simulink model "OnePhInverterRL_17b"  (R2020a)
settings: Solver=ode23tb  StartTime=0.0  StopTime=1  MaxStep=2e-3  RelTol=1e-3
model workspace (MAT data in the model file):
  TLoad = [0.005 0.1]
libraries: powerlib x15, powerlib_meascontrol x9
settings Model: Creator=theo  LastModifiedBy=Theodore
settings DebuggingCC: ArithmeticOperatorsInVariantConditions=warning
settings SFSimCC: CustomCodeUndefinedFunction=UseInterfaceOnly

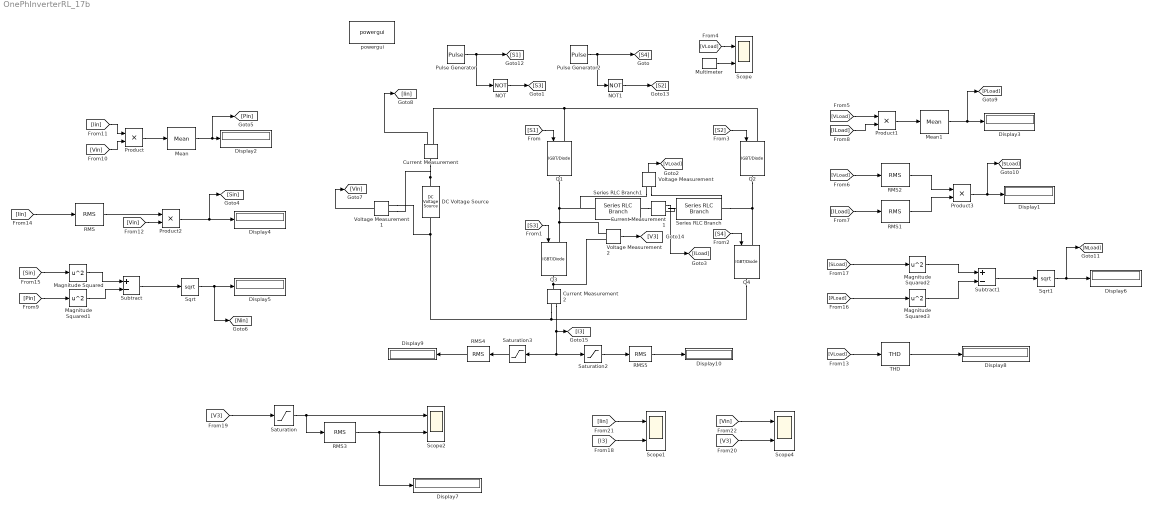
== system OnePhInverterRL_17b ==
  Current Measurement : powerlib/Measurements/Current Measurement  PhasorSimulation=off  OutputType=Complex  PSBequivalent=0
  Current Measurement1 : powerlib/Measurements/Current Measurement  PhasorSimulation=off  OutputType=Complex  PSBequivalent=0
  Current Measurement2 : powerlib/Measurements/Current Measurement  PhasorSimulation=off  OutputType=Complex  PSBequivalent=0
  DC Voltage Source : powerlib/Electrical Sources/DC Voltage Source  Amplitude=537.97  Measurements=None
  Display{1..10} (10 alike) : Display
  Magnitude Squared{,1..3} (4 alike) : Math  Operator=square  SaturateOnIntegerOverflow=on
  Mean : powerlib_meascontrol/Measurements/Mean  Freq=50  Vinit=0  Ts=0
  Mean1 : powerlib_meascontrol/Measurements/Mean  Freq=50  Vinit=0  Ts=0
  Multimeter : powerlib/Measurements/Multimeter  PhasorSimulation=off  OutputType=Complex  sel=2  L=2  Gain=1  yselected={'Ib: Series RLC Branch1'};  PSBOutputType=1  PSBequivalent=0  AxesSetting=[0,0.1,-100,100]  Display=0  SavedBlockNames=-11
  NOT : Logic  Operator=NOT  IconShape=distinctive  AllPortsSameDT=off  OutDataTypeStr=boolean
  NOT1 : Logic  Operator=NOT  IconShape=distinctive  AllPortsSameDT=off  OutDataTypeStr=boolean
  Product{,1..3} (4 alike) : Product
  Pulse Generator : DiscretePulseGenerator  PulseType=Time based  Period=0.02  PulseWidth=50
  Pulse Generator2 : DiscretePulseGenerator  PulseType=Time based  Period=0.02  PulseWidth=50
  Q{1..4} (4 alike) : powerlib/Power Electronics/IGBT//Diode  Ron=1e-3  Rs=1e5  Cs=inf  Measurements=off
  RMS{,1..5} (6 alike) : powerlib_meascontrol/Measurements/RMS  TrueRMS=on  Freq=50  RMSInit=120  Ts=0
  Saturation : Saturate  UpperLimit=0  LowerLimit=-50
  Saturation2 : Saturate  UpperLimit=0  LowerLimit=-100
  Saturation3 : Saturate  UpperLimit=100  LowerLimit=0
  Scope{,1..2,4} (4 alike) : Scope  NumInputPorts=2
  Series RLC Branch : powerlib/Elements/Series RLC Branch  LConnTagsString=__new0  RConnTagsString=__new0  BranchType=L  Resistance=10  Inductance=1/(2*pi)  SetiL0=off  InitialCurrent=0  Capacitance=1e-6  Setx0=off  InitialVoltage=0  Measurements=None
  Series RLC Branch1 : powerlib/Elements/Series RLC Branch  LConnTagsString=__new0  RConnTagsString=__new0  BranchType=R  Resistance=50  Inductance=1e-3  SetiL0=off  InitialCurrent=0  Capacitance=1e-6  Setx0=off  InitialVoltage=0  Measurements=Branch voltage and current
  Sqrt : Sqrt  SaturateOnIntegerOverflow=on
  Sqrt1 : Sqrt  SaturateOnIntegerOverflow=on
  Subtract : Sum  Inputs=+-
  Subtract1 : Sum  Inputs=+-
  THD : powerlib_meascontrol/Measurements/THD  Freq=50  Ts=0
  Voltage Measurement : powerlib/Measurements/Voltage Measurement  PhasorSimulation=off  OutputType=Complex  PSBequivalent=0
  Voltage Measurement1 : powerlib/Measurements/Voltage Measurement  PhasorSimulation=off  OutputType=Complex  PSBequivalent=0
  Voltage Measurement2 : powerlib/Measurements/Voltage Measurement  PhasorSimulation=off  OutputType=Complex  PSBequivalent=0
  powergui : powerlib/powergui  Priority=1  SimulationMode=Continuous  SampleTime=50e-6  frequency=50  Iterations=50  frequencyindice=0  Pbase=100e6  ErrMax=1e-4  UnitsV=kV  UnitsW=MW  buscounter=0  FunctionMessages=off  echomessages=off  EnableUseOfTLC=off  CurrentSourceSwitches=off  DisableSnubberDevices=on  DisableRonSwitches=on  DisableVfSwitches=on  DisplayEquations=off  AutomaticDiscreteSolvers=off  SolverType=Tustin/Backward Euler (TBE)  Interpol=off  ExternalGateDelay=off  methode=off  Ts=100  x0status=blocks  SPID=on  SwTol=0  HookPort=off  NonlinearTolerance=1e-4  nMaxIteration=100  ContinueOnMaxIteration=off  RestoreLinks=warning  ResistiveCurrentMeasurement=off  Frange=[0:2:500]  Ylog=off  Xlog=on  ShowGrid=off  save=off  variable=ZData  structure=0  ZoomFFT=off  StartTime=0.0  cycles=1  DisplayStyle=1  fundamental=60  FreqAxis=off  MaxFrequency=1000  frequencyindicesteady=1  RmsSteady=1  display=off
  wires:
  Pulse Generator/1 -> NOT/1, [S1]
  NOT/1 -> [S3]
  [S1] -> Q1/1
  [S4] -> Q4/1
  [S3] -> Q3/1
  [S2] -> Q2/1
  Voltage Measurement/1 -> [VLoad]
  [VLoad] -> Scope/1
  Multimeter/1 -> Scope/2
  Current Measurement/1 -> [Iin]
  Product/1 -> Mean/1
  Mean/1 -> [Pin], Display2/1
  Voltage Measurement1/1 -> [Vin]
  [VLoad] -> Product1/1
  Product1/1 -> Mean1/1
  Mean1/1 -> [PLoad], Display3/1
  RMS/1 -> Product2/1
  Product2/1 -> [Sin], Display4/1
  RMS2/1 -> Product3/1
  RMS1/1 -> Product3/2
  Current Measurement1/1 -> [ILoad]
  [ILoad] -> RMS1/1
  [VLoad] -> RMS2/1
  [ILoad] -> Product1/2
  Magnitude Squared/1 -> Subtract/1
  Magnitude Squared1/1 -> Subtract/2
  Subtract/1 -> Sqrt/1
  Sqrt/1 -> [Nin], Display5/1
  Subtract1/1 -> Sqrt1/1
  Product3/1 -> [SLoad], Display1/1
  Magnitude Squared2/1 -> Subtract1/1
  Magnitude Squared3/1 -> Subtract1/2
  Sqrt1/1 -> [NLoad], Display6/1
  [Vin] -> Product/2
  [Vin] -> Product2/2
  [Iin] -> Product/1
  [Iin] -> RMS/1
  [Pin] -> Magnitude Squared1/1
  [Sin] -> Magnitude Squared/1
  [PLoad] -> Magnitude Squared3/1
  [SLoad] -> Magnitude Squared2/1
  Pulse Generator2/1 -> [S4], NOT1/1
  NOT1/1 -> [S2]
  [VLoad] -> THD/1
  THD/1 -> Display8/1
  [V3] -> Saturation/1
  Saturation/1 -> Scope2/1, RMS3/1
  RMS3/1 -> Display7/1, Scope2/2
  Voltage Measurement2/1 -> [V3]
  Current Measurement2/1 -> [I3], Saturation3/1, Saturation2/1
  RMS4/1 -> Display9/1
  RMS5/1 -> Display10/1
  Saturation2/1 -> RMS5/1
  Saturation3/1 -> RMS4/1
  [Vin] -> Scope4/1
  [Iin] -> Scope1/1
  [V3] -> Scope4/2
  [I3] -> Scope1/2
  connections:
  Q1/RConn1 -- Voltage Measurement/LConn1 -- Series RLC Branch1/LConn1 -- Voltage Measurement2/LConn1 -- Q3/LConn1
  Q2/RConn1 -- Voltage Measurement/LConn2 -- Series RLC Branch/RConn1 -- Q4/LConn1
  Q4/RConn1 -- Current Measurement2/RConn1 -- Voltage Measurement1/LConn2 -- DC Voltage Source/LConn1
  DC Voltage Source/RConn1 -- Current Measurement/LConn1 -- Voltage Measurement1/LConn1
  Q2/LConn1 -- Q1/LConn1 -- Current Measurement/RConn1
  Series RLC Branch1/RConn1 -- Current Measurement1/LConn1
  Series RLC Branch/LConn1 -- Current Measurement1/RConn1
  Q3/RConn1 -- Current Measurement2/LConn1 -- Voltage Measurement2/LConn2
